simulink model "QAM_Mod_with_Dmod"  (R2022a)
settings: Solver=VariableStepAuto  StartTime=0.0  StopTime=1000  RelTol=1e-3
undefined symbols (not defined in the file): xc7s100fgga676
libraries: hdlBasic x18, commrandsrc3 x1, vmcUtilities x1
settings Model: Creator=Sandesh  LastModifiedBy=Sandesh

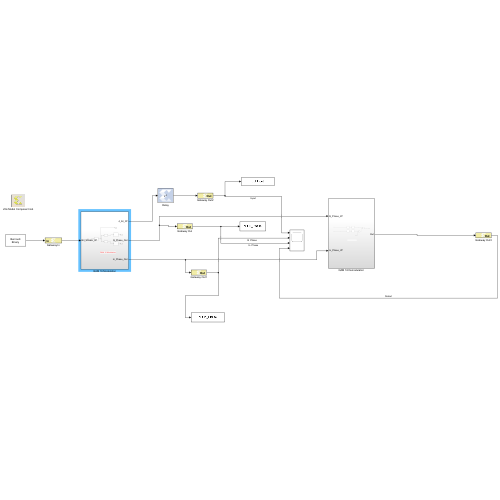
[thumbnail: Simulink's stored preview of the top-level diagram]
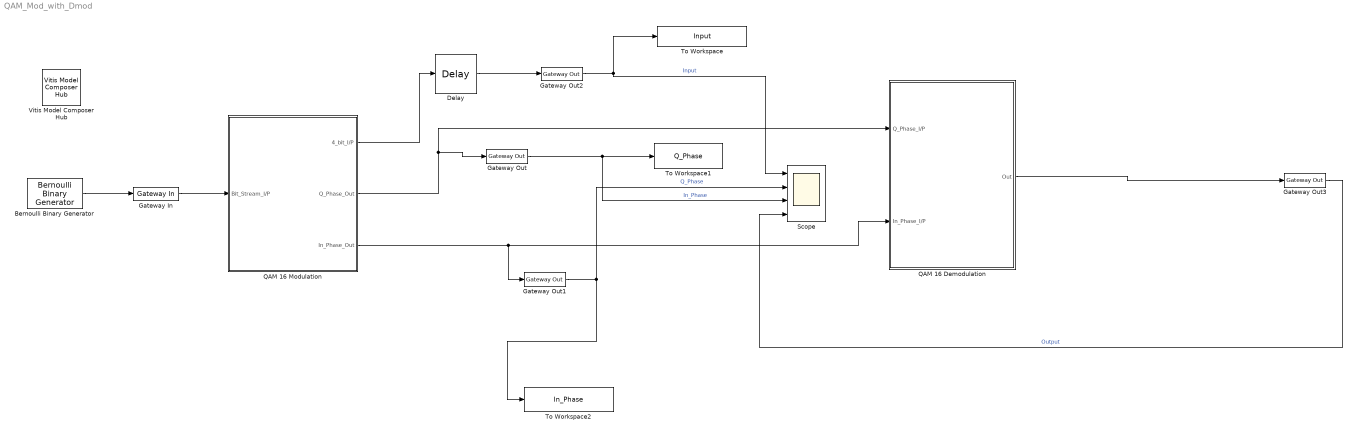
== system QAM_Mod_with_Dmod ==
  Bernoulli Binary Generator : commrandsrc3/Bernoulli Binary Generator  ProbabilityOfZero=0.5  SeedSource=Auto  Seed=0  SampleTime=1  SamplesPerFrame=1  OutputDataType=double  SimulateUsing=Interpreted execution
  Delay : hdlBasic/Delay  rst=off  en=off  latency=2  reg_retiming=off  XmcBlockStatus=1  maskContainerNames=group1  block_type=delay  block_config=sysgen:Delay_config
  Gateway In : hdlBasic/Gateway In  gui_display_data_type=Fixed-point  arith_type=Unsigned  n_bits=1  bin_pt=0  preci_type=Single  exp_width=8  frac_width=24  rows=1  columns=1  quantization="Round  (unbiased: +/- Inf)"  overflow=Saturate  period=1  UseAsADC=off  ADCChannel='1'  interface=None  automatic_assignment=on  address_offset=hex2dec('00')  intf_name=''  intf_description=''  default_value=0  timing_constraint=None  locs_specified=off  LOCs={}  io_standard={}  inherit_from_input=off  hdl_port=on  XmcBlockStatus=1  maskContainerNames=group4  block_type=gatewayin  block_config=sysgen:gateway_in_config  block_width_w=590  block_height_w=620  block_width=640  block_height=850
  Gateway Out{,1..3} (4 alike) : hdlBasic/Gateway Out  inherit_from_input=off  hdl_port=on  rows=1  columns=1  UseAsDAC=off  DACChannel='1'  interface=None  automatic_assignment=on  address_offset=hex2dec('00')  intf_name=''  intf_description=''  timing_constraint=None  locs_specified=off  LOCs={}  io_standard={}  XmcBlockStatus=1  maskContainerNames=group4  block_type=gatewayout  block_config=sysgen:gateway_out_config  block_width_w=590  block_height_w=620  block_width=620  block_height=750
  QAM 16 Demodulation : Subsystem
  QAM 16 Modulation : Subsystem
  Scope : Scope  NumInputPorts=4
  To Workspace : ToWorkspace  VariableName=Input  SaveFormat=Timeseries  SampleTime=-1
  To Workspace1 : ToWorkspace  VariableName=Q_Phase  SaveFormat=Timeseries  SampleTime=-1
  To Workspace2 : ToWorkspace  VariableName=In_Phase  SaveFormat=Timeseries  SampleTime=-1
  Vitis Model Composer Hub : vmcUtilities/Vitis Model Composer Hub  Tag=genX  CodeGeneration=off  TargetDirectory=./code  ExportType=AI Engines  IpVendor=xilinx.com  IpLibrary=hls  IpVersion=1.0  IpHWLanguage=Verilog  AieCompilerOptions={}  CreateTestbench=off  TestbenchStackSize=10  RunAieSim=off  AieSimTimeout=50000  RunAieSimProfiling=off  LaunchVitisAnalyzer=off  PlotOutput=off  RunX86Sim=off  X86SimTimeout=10  GenHwImage=off  PlatformType=Not Specified  HwSystemType=Baremetal  HwValidationTarget=hw  ProjDevice=Spartan-7 SP701 Evaluation Platform (xc7s100fgga676-2)  ProjDevicePart=xc7s100fgga676-2  SamplePeriod=-1  ClockFrequency=200  DataPathParallelism=1  xilinxfamily=spartan7  part=xc7s100  speed=-2  package=fgga676  directory=./netlist  testbench=off  incr_netlist=off  synthesis_tool=Vivado  clock_wrapper=Clock Enables  dbl_ovrd=According to Block Masks  dcm_input_clock_period=10  sysclk_period=10  simulink_period=1  eval_field=0
  wires:
  Gateway Out1/1 -> Scope/2, To Workspace2/1  "Q_Phase"
  Gateway Out/1 -> Scope/3, To Workspace1/1  "In_Phase"
  Gateway Out2/1 -> To Workspace/1, Scope/1  "Input"
  Bernoulli Binary Generator/1 -> Gateway In/1
  Gateway Out3/1 -> Scope/4  "Output"
  QAM 16 Modulation/2(Q_Phase_Out) -> QAM 16 Demodulation/1(Q_Phase_I/P), Gateway Out/1
  QAM 16 Modulation/3(In_Phase_Out) -> QAM 16 Demodulation/2(In_Phase_I/P), Gateway Out1/1
  Gateway In/1 -> QAM 16 Modulation/1(Bit_Stream_I/P)
  QAM 16 Modulation/1(4_bit_I/P) -> Delay/1
  QAM 16 Demodulation/1(Out) -> Gateway Out3/1
  Delay/1 -> Gateway Out2/1

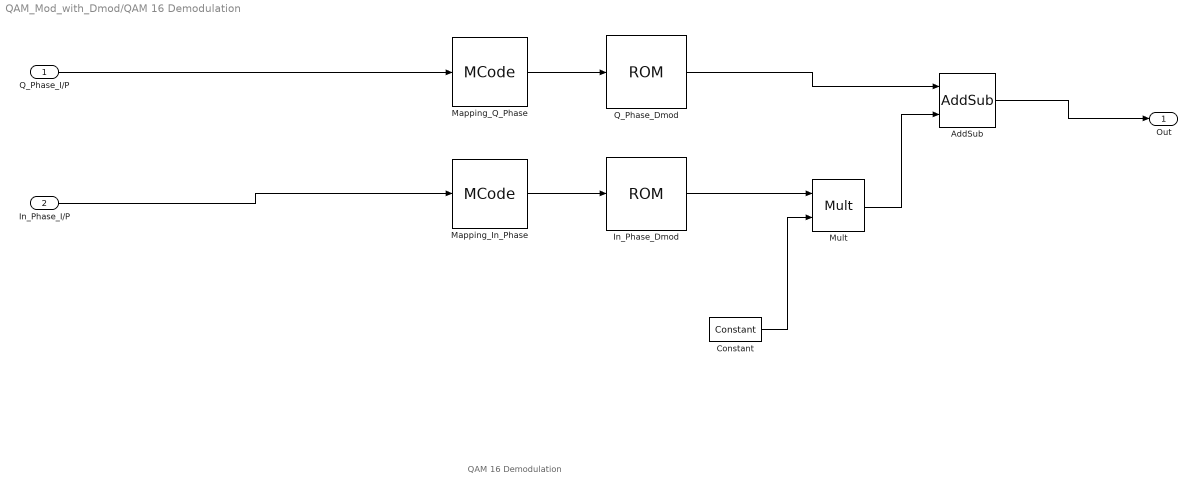
== system QAM_Mod_with_Dmod/QAM 16 Demodulation ==
  note: QAM 16 Demodulation
  Q_Phase_I/P : Inport
  In_Phase_I/P : Inport  Port=2
  AddSub : hdlBasic/AddSub  mode=Addition  use_carryin=off  use_carryout=off  en=off  latency=0  precision=Full  arith_type=Unsigned  n_bits=16  bin_pt=14  quantization=Truncate  overflow=Wrap  use_behavioral_HDL=off  hw_selection=Fabric  pipelined=off  XmcBlockStatus=1  maskContainerNames=tabcontainer1  block_type=addsub  block_config=sysgen:Addsub_config
  Constant : hdlBasic/Constant  const=4  gui_display_data_type=Fixed-point  arith_type=Unsigned  n_bits=4  bin_pt=0  preci_type=Single  exp_width=8  frac_width=24  explicit_period=off  period=1  XmcBlockStatus=1  maskContainerNames=tabcontainer1  block_type=constant  block_config=sysgen:Constant_config
  In_Phase_Dmod : hdlBasic/ROM  depth=4  initVector=[0 1 2 3]  distributed_mem=Block RAM  rst=off  init_reg=0  en=off  latency=1  gui_display_data_type=Fixed-point  arith_type=Unsigned  n_bits=2  bin_pt=0  preci_type=Double  exp_width=8  frac_width=24  optimize=Area  use_rpm=on  simulation_type=fast_sim  XmcBlockStatus=1  maskContainerNames=tabcontainer1  block_type=sprom  block_config=sysgen:SPROM_config
  Mapping_In_Phase : hdlBasic/MCode  mfname=Mapping  explicit_period=off  period=1  iptable={ 'I', '' }  optable={ 'B', 'off' }  enable_stdout=off  enable_debug=off  suppress_output='on'  defparams={}  hide_port_list={}  block_type=mcode  block_width=444  block_height=788
      settings: infoedit=Pass input values to a MATLAB function for evaluation in Xilinx fixed-point type. The input ports of the block are input arguments of the function. The output ports of the block are output arguments of the function.
  Mapping_Q_Phase : hdlBasic/MCode  mfname=Mapping  explicit_period=off  period=1  iptable={ 'I', '' }  optable={ 'B', 'off' }  enable_stdout=off  enable_debug=off  suppress_output='on'  defparams={}  hide_port_list={}  block_type=mcode  block_width=444  block_height=788
      settings: infoedit=Pass input values to a MATLAB function for evaluation in Xilinx fixed-point type. The input ports of the block are input arguments of the function. The output ports of the block are output arguments of the function.
  Mult : hdlBasic/Mult  precision=Full  arith_type=Unsigned  n_bits=4  bin_pt=14  quantization=Truncate  overflow=Wrap  en=off  latency=0  use_behavioral_HDL=off  opt=Speed  use_embedded=on  optimum_pipeline=off  pipeline=on  use_rpm=on  placement_style=Triangular  XmcBlockStatus=1  maskContainerNames=group1  block_type=mult  block_config=sysgen:Mult_config  block_width=598  block_height=876
  Q_Phase_Dmod : hdlBasic/ROM  depth=4  initVector=[3 2 1 0]  distributed_mem=Block RAM  rst=off  init_reg=0  en=off  latency=1  gui_display_data_type=Fixed-point  arith_type=Unsigned  n_bits=2  bin_pt=0  preci_type=Double  exp_width=8  frac_width=24  optimize=Area  use_rpm=on  simulation_type=fast_sim  XmcBlockStatus=1  maskContainerNames=tabcontainer1  block_type=sprom  block_config=sysgen:SPROM_config
  Out : Outport
  wires:
  Mapping_In_Phase/1 -> In_Phase_Dmod/1
  Mapping_Q_Phase/1 -> Q_Phase_Dmod/1
  In_Phase_I/P/1 -> Mapping_In_Phase/1
  Q_Phase_I/P/1 -> Mapping_Q_Phase/1
  In_Phase_Dmod/1 -> Mult/1
  Mult/1 -> AddSub/2
  Constant/1 -> Mult/2
  AddSub/1 -> Out/1
  Q_Phase_Dmod/1 -> AddSub/1

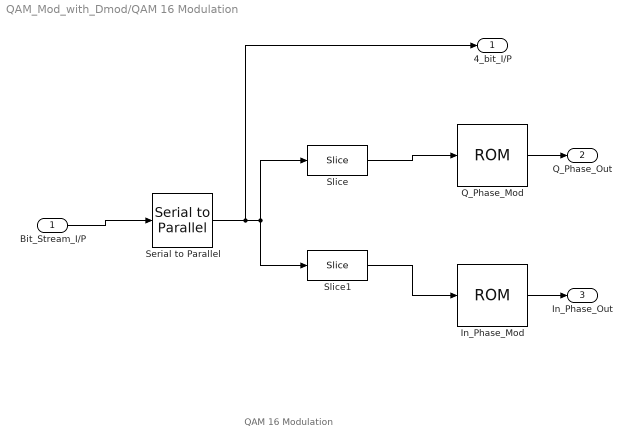
== system QAM_Mod_with_Dmod/QAM 16 Modulation ==
  note: QAM 16 Modulation
  Bit_Stream_I/P : Inport
  In_Phase_Mod : hdlBasic/ROM  depth=4  initVector=[-3 -1 +1 +3]  distributed_mem=Block RAM  rst=off  init_reg=0  en=off  latency=1  gui_display_data_type=Fixed-point  arith_type="Signed  (2's comp)"  n_bits=16  bin_pt=13  preci_type=Single  exp_width=8  frac_width=24  optimize=Area  use_rpm=on  simulation_type=fast_sim  XmcBlockStatus=1  maskContainerNames=tabcontainer1  block_type=sprom  block_config=sysgen:SPROM_config
  Q_Phase_Mod : hdlBasic/ROM  depth=4  initVector=[+3 +1 -1 -3]  distributed_mem=Block RAM  rst=off  init_reg=0  en=off  latency=1  gui_display_data_type=Fixed-point  arith_type="Signed  (2's comp)"  n_bits=16  bin_pt=13  preci_type=Single  exp_width=8  frac_width=24  optimize=Area  use_rpm=on  simulation_type=fast_sim  XmcBlockStatus=1  maskContainerNames=tabcontainer1  block_type=sprom  block_config=sysgen:SPROM_config
  Serial to Parallel : hdlBasic/Serial to Parallel  input_order=Least Significant Word First  arith_type=Unsigned  output_bits=4  bin_pt=0  rst=off  en=off  latency=1  input_bits=[]  XmcBlockStatus=1  maskContainerNames=group3  block_type=s2p  block_config=sysgen:S2P_config
  Slice : hdlBasic/Slice  nbits=2  boolean_output=off  mode=Lower Bit Location + Width  bit1=0  base1=MSB of Input  bit0=0  base0=LSB of Input  XmcBlockStatus=1  maskContainerNames=group1  block_type=slice  block_config=sysgen:Slice_config
  Slice1 : hdlBasic/Slice  nbits=2  boolean_output=off  mode=Upper Bit Location + Width  bit1=0  base1=MSB of Input  bit0=0  base0=LSB of Input  XmcBlockStatus=1  maskContainerNames=group1  block_type=slice  block_config=sysgen:Slice_config
  4_bit_I/P : Outport
  Q_Phase_Out : Outport  Port=2
  In_Phase_Out : Outport  Port=3
  wires:
  Serial to Parallel/1 -> 4_bit_I/P/1, Slice/1, Slice1/1
  Q_Phase_Mod/1 -> Q_Phase_Out/1
  Slice/1 -> Q_Phase_Mod/1
  Slice1/1 -> In_Phase_Mod/1
  Bit_Stream_I/P/1 -> Serial to Parallel/1
  In_Phase_Mod/1 -> In_Phase_Out/1
